simulink model "appKnbSwt"  (R2025b)
settings: Solver=FixedStepAuto  StartTime=0.0  StopTime=10.0  FixedStep=0.01  RelTol=1e-3
PostLoadFcn:
  | % Automatically enforce bare-metal code generation rules on model load
  | set_param(bdroot, 'IncludeMdlTerminateFcn', 'off');
  | set_param(bdroot, 'RemoveResetFunc', 'on');
  | set_param(bdroot, 'RemoveDisableFunc', 'on');
values from neighbouring files (symbols this model uses):
  ADC_MAX = 1023.0    [appKnbSwt.sldd]
  Knb_Hyst_Pc_Pt = 5.0    [appKnbSwt.sldd]
  Knb_Thresh_Pc_Pt = 20.0    [appKnbSwt.sldd]
  PCT_MAX = 100.0    [appKnbSwt.sldd]
settings Model: DataDictionary=appKnbSwt.sldd  Creator=eren  LastModifiedBy=eren
settings OptimizationCC: DefaultParameterBehavior=Inlined  UseDivisionForNetSlopeComputation=on  GainParamInheritBuiltInType=on  UseFloatMulNetSlope=on  InlineInvariantSignals=on  EnhancedBackFolding=on  BooleansAsBitfields=on  PassReuseOutputArgsAs=Individual arguments  StateBitsets=on  DataBitsets=on  ZeroExternalMemoryAtStartup=off  ZeroInternalMemoryAtStartup=off  NoFixptDivByZeroProtection=on  EfficientFloat2IntCast=on  LifeSpan=1  OptimizeBlockOrder=speed  DifferentSizesBufferReuse=on  EfficientTunableParamExpr=on
settings DebuggingCC: ParameterTunabilityLossMsg=error
settings HardwareCC: ProdBitPerInt=16.0  ProdBitPerPointer=16.0  ProdBitPerSizeT=16.0  ProdBitPerPtrDiffT=16.0  ProdLargestAtomicFloat=None  ProdWordSize=16.0  ProdHWDeviceType=Atmel->AVR (8-bit)
settings SFSimCC: MATLABDynamicMemAlloc=off
settings RTWCC: SystemTargetFile=ert.tlc  GenCodeOnly=on  TemplateMakefile=ert_default_tmf  Description=Embedded Coder
settings CodeAppCC: ForceParamTrailComments=on  IgnoreCustomStorageClasses=off  OperatorAnnotations=on  SimulinkDataObjDesc=on  SFDataObjDesc=on  CustomSymbolStrGlobalVar=rt$N$M  CustomSymbolStrType=$N$M  CustomSymbolStrFcn=$N$M$F  CustomSymbolStrMacro=$N$M  InsertBlockDesc=on
settings ERTTargetCC: ERTCustomFileTemplate=example_file_process.tlc  ERTFilePackagingFormat=CompactWithDataFile  TargetLangStandard=C99 (ISO)  IncludeMdlTerminateFcn=off  CombineSignalStateStructs=on  SupportAbsoluteTime=off  PurelyIntegerCode=on  SupportNonFinite=off  SupportComplex=off  RemoveDisableFunc=on

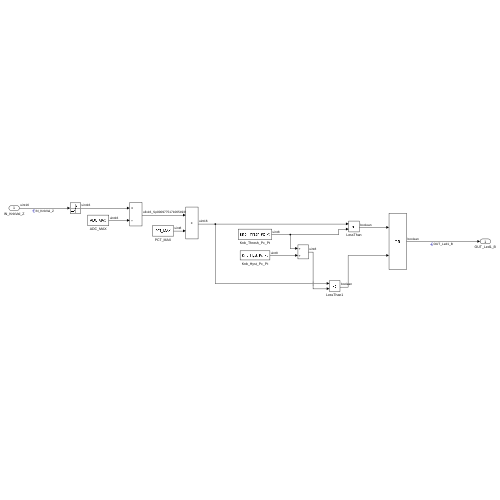
[thumbnail: Simulink's stored preview of the top-level diagram]
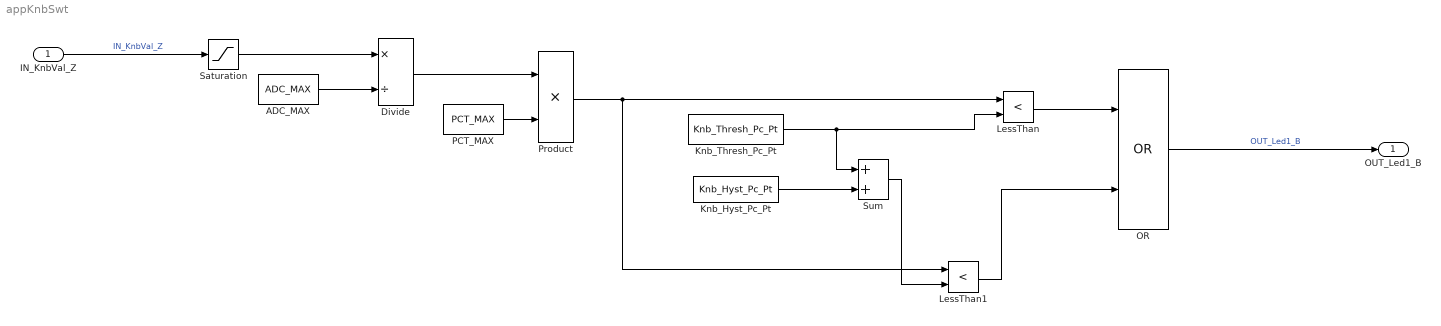
== system appKnbSwt ==
  IN_KnbVal_Z : Inport
  ADC_MAX : Constant  Value=ADC_MAX
  Divide : Product  Inputs=*/  OutDataTypeStr=DT_Ratio  SaturateOnIntegerOverflow=on
  Knb_Hyst_Pc_Pt : Constant  Value=Knb_Hyst_Pc_Pt
  Knb_Thresh_Pc_Pt : Constant  Value=Knb_Thresh_Pc_Pt
  LessThan : RelationalOperator  Operator=<  OutDataTypeStr=boolean  RndMeth=Simplest  InputSameDT=off
  LessThan1 : RelationalOperator  Operator=<  OutDataTypeStr=boolean  RndMeth=Simplest  InputSameDT=off
  OR : Logic  Operator=OR  AllPortsSameDT=off  OutDataTypeStr=boolean
  PCT_MAX : Constant  Value=PCT_MAX
  Product : Product  OutDataTypeStr=uint16  SaturateOnIntegerOverflow=on
  Saturation : Saturate  UpperLimit=1023  LowerLimit=0
  Sum : Sum  InputSameDT=on  SaturateOnIntegerOverflow=on
  OUT_Led1_B : Outport
  wires:
  ADC_MAX/1 -> Divide/2
  IN_KnbVal_Z/1 -> Saturation/1  "IN_KnbVal_Z"
  Divide/1 -> Product/1
  PCT_MAX/1 -> Product/2
  Product/1 -> LessThan1/1, LessThan/1
  Knb_Hyst_Pc_Pt/1 -> Sum/2
  Knb_Thresh_Pc_Pt/1 -> Sum/1, LessThan/2
  LessThan/1 -> OR/1
  LessThan1/1 -> OR/2
  OR/1 -> OUT_Led1_B/1  "OUT_Led1_B"
  Sum/1 -> LessThan1/2
  Saturation/1 -> Divide/1
